simulink model "CarSim_SCANeR_UDP_ACC_THESIS"  (R2019a)
settings: Solver=FixedStepAuto  StartTime=0.0  StopTime=inf  FixedStep=0.001  RelTol=1e-3  EnableMultiTasking=on
undefined symbols (not defined in the file or in its folder): DWORK0, DWORK1
libraries: simulink x14, xpcutilitieslib x2, xpcrtudplib x2, dspnetwork x1
(part 1 of 2)
settings Model: ExtModeTrigDuration=10000  Creator=llacroix  LastModifiedBy=wilkerson.102
settings SolverCC: PositivePriorityOrder=on  InsertRTBMode=Always
settings DataIOCC: ReturnWorkspaceOutputs=off
settings OptimizationCC: UseFloatMulNetSlope=on
settings DebuggingCC: ArithmeticOperatorsInVariantConditions=warning
settings SFSimCC: SimUseLocalCustomCode=off
settings RTWCC: Description=Generic Real-Time Target  RTWUseLocalCustomCode=off  TargetLang=C++
settings CodeAppCC: StateflowObjectComments=on
settings GRTTargetCC: TargetLangStandard=C++03 (ISO)  MatFileLogging=off  MultiInstanceERTCode=on  CodeInterfacePackaging=C++ class

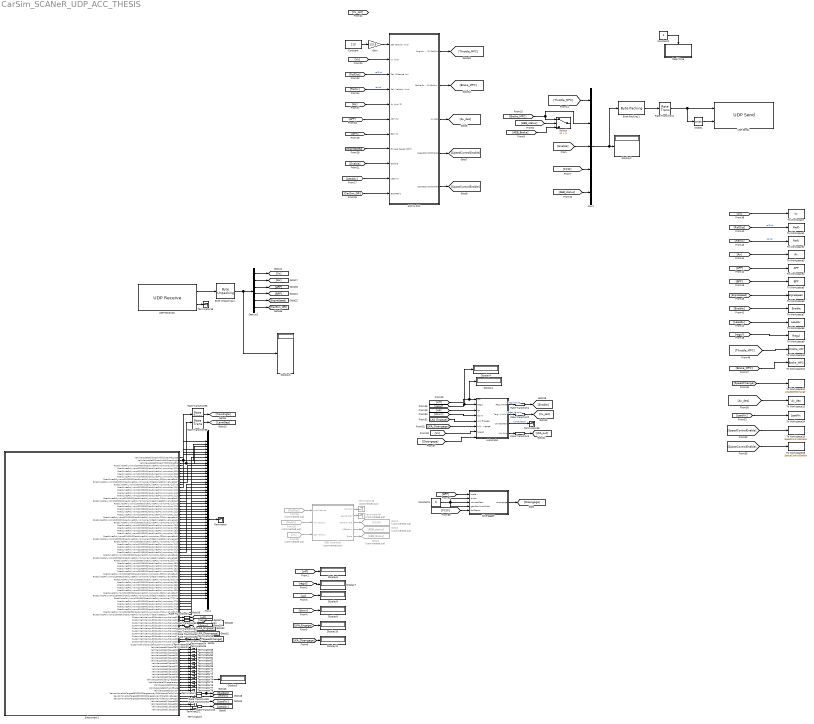
== system CarSim_SCANeR_UDP_ACC_THESIS ==
  ACC & CC1 : Subsystem
  AEB Controller : Subsystem  Commented=on
  Automate : Subsystem
  Byte Packing 1 : xpcutilitieslib/Byte Packing   MaskPackedDataType=uint8  MaskUnpackedDataTypes={'double'}  MaskAlignment=1
  Byte Unpacking 2 : xpcutilitieslib/Byte Unpacking   MaskUnpackedDataTypes={'double'}  MaskUnpackedDataSizes={[6]}  MaskAlignment=1
      settings: SourceProductName=Simulink Real-Time  SourceProductBaseCode=XP
  Constant : Constant  Value=110  VectorParams1D=off
  Constant1 : Constant  Value=0
  Constant2 : Constant
  Demux2 : Demux  Outputs=6
  Disengager : Subsystem
  Display{1..11} (11 alike) : Display
  From16 : From  Commented=on  GotoTag=RelDist
  From35 : From  Commented=on  GotoTag=RelVx
  From36 : From  Commented=on  GotoTag=Vx
  Gain : Gain  Gain=1/3.6
  Goto1 : Goto  Commented=on  GotoTag=FCW
  Goto2 : Goto  Commented=on  GotoTag=AEB_status
  Goto3 : Goto  Commented=on  GotoTag=AEB_Brake
  Mux1 : Mux  Inputs=5
  Mux4 : Mux  Inputs=59
  Rate Transition{1..5,55..64} (15 alike) : RateTransition
  Real-Time : Subsystem
  Subsystem1 : Subsystem
  Switch : Switch  Criteria=u2 > Threshold
  Terminator{,1..3,18,23,53..63,68..78} (28 alike) : Terminator
  Terminator48 : Terminator  Commented=on
  Terminator49 : Terminator  Commented=on
  To Workspace : ToWorkspace  VariableName=Vx  SampleTime=-1
      settings: Save2DSignal=2-D array (concatenate along first dimension)
  To Workspace1 : ToWorkspace  VariableName=RelD  SampleTime=-1
      settings: Save2DSignal=2-D array (concatenate along first dimension)
  To Workspace10 : ToWorkspace  VariableName=Throttle_MPC  SampleTime=-1
      settings: Save2DSignal=2-D array (concatenate along first dimension)
  To Workspace11 : ToWorkspace  VariableName=Brake_MPC  SampleTime=-1
      settings: Save2DSignal=2-D array (concatenate along first dimension)
  To Workspace12 : ToWorkspace  VariableName=LeadSpeedChange  SampleTime=-1
      settings: Save2DSignal=2-D array (concatenate along first dimension)
  To Workspace13 : ToWorkspace  VariableName=Ax_des  SampleTime=-1
      settings: Save2DSignal=2-D array (concatenate along first dimension)
  To Workspace14 : ToWorkspace  VariableName=LeadVx  SampleTime=-1
      settings: Save2DSignal=2-D array (concatenate along first dimension)
  To Workspace15 : ToWorkspace  VariableName=SpeedControlEnable  SampleTime=-1
      settings: Save2DSignal=2-D array (concatenate along first dimension)
  To Workspace16 : ToWorkspace  VariableName=SpaceControlEnable  SampleTime=-1
      settings: Save2DSignal=2-D array (concatenate along first dimension)
  To Workspace2 : ToWorkspace  VariableName=RelV  SampleTime=-1
      settings: Save2DSignal=2-D array (concatenate along first dimension)
  To Workspace3 : ToWorkspace  VariableName=Ax  SampleTime=-1
      settings: Save2DSignal=2-D array (concatenate along first dimension)
  To Workspace4 : ToWorkspace  VariableName=APP  SampleTime=-1
      settings: Save2DSignal=2-D array (concatenate along first dimension)
  To Workspace5 : ToWorkspace  VariableName=BPP  SampleTime=-1
      settings: Save2DSignal=2-D array (concatenate along first dimension)
  To Workspace6 : ToWorkspace  VariableName=EngineSpeed  SampleTime=-1
      settings: Save2DSignal=2-D array (concatenate along first dimension)
  To Workspace7 : ToWorkspace  VariableName=Enable  SampleTime=-1
      settings: Save2DSignal=2-D array (concatenate along first dimension)
  To Workspace8 : ToWorkspace  VariableName=LeadAx  SampleTime=-1
      settings: Save2DSignal=2-D array (concatenate along first dimension)
  To Workspace9 : ToWorkspace  VariableName=Regul  SampleTime=-1
      settings: Save2DSignal=2-D array (concatenate along first dimension)
  UDP Receive2 : xpcrtudplib/UDP Receive  ipAddressVal=Use host-target connection  localPort=25007  rcvWidth=48  rcvFmAny=off  fmAddress=0.0.0.0  rcvMulticast=off  multicastAddress={}  maxUDPQueue=8  sampleTime=0.001
      settings: SourceProductName=Simulink Real-Time
  UDP Send1 : xpcrtudplib/UDP Send  ipAddressVal=Use host-target connection  localPort=-1  toAddress=255.255.255.255  toPort=25004  sampleTime=0.01
      settings: SourceProductName=Simulink Real-Time  SourceProductBaseCode=XP
  Width1 : Width
  wires:
  Automate/2(Target (m/s)) -> Rate Transition2/1  "Target Velocity"
  Automate/1(RegulMode) -> Rate Transition1/1  "RegulMode"
  Automate/3(wantedGear) -> Terminator68/1  "wantedGear"
  Automate/4(LKA Out) -> Rate Transition3/1
  Rate Transition1/1 -> [Enable]
  Rate Transition2/1 -> [Vx_set]
  Rate Transition3/1 -> [LKA_out]
  [off] -> Display1/1, Automate/1(Off)
  [regul] -> Display4/1, Automate/2(Regul)
  [up] -> Automate/3(Up)
  [down] -> Automate/4(Down)
  [LKA_Engage] -> Automate/5(LKA Engage)
  [LKA_Disengage] -> Automate/6(LKA Disengage)
  [Vx] -> Automate/7(Speed)
  [Disengage] -> Automate/8(disengage)
  Rate Transition4/1 -> UDP Send1/1, Width1/1
  Byte Packing 1/1 -> Rate Transition4/1
  Width1/1 -> UDP Send1/2
  [Vx] -> ACC & CC1/2(Vx (m/s))
  [RelDist] -> ACC & CC1/3(Rel. Distance (m))  "relDist"
  [RelVx] -> ACC & CC1/4(Rel. Velocity (m/s))  "relVel"
  [Ax] -> ACC & CC1/5(Ax (m/s^2))
  [APP] -> ACC & CC1/6(APP (%))
  [BPP] -> ACC & CC1/7(BPP (N))
  [EngineSpeed] -> ACC & CC1/8(Eninge Speed (RPM))
  [Enable] -> ACC & CC1/9(Enable)
  [LeadAx] -> ACC & CC1/10(Lead Ax)
  [CarSim_GR] -> ACC & CC1/11(GearRatio)
  ACC & CC1/2(Brake Force (N) CarSim) -> [Brake_MPC]
  ACC & CC1/1(Engine Throttle (%) CarSim) -> [Throttle_MPC]
  Mux1/1 -> Byte Packing 1/1, Display2/1
  [Throttle_MPC] -> Mux1/1
  UDP Receive2/1 -> Byte Unpacking 2/1
  UDP Receive2/2 -> Terminator18/1
  Byte Unpacking 2/1 -> Display3/1, Demux2/1
  Demux2/1 -> [Vx]
  Demux2/2 -> [Ax]
  Demux2/3 -> [APP]
  Demux2/4 -> [BPP]
  Demux2/5 -> [EngineSpeed]
  Demux2/6 -> [CarSim_GR]
  [BPP] -> Disengager/1(brake)
  Constant1/1 -> Disengager/2(clutch), Disengager/4(gearBoxAutoMode), Disengager/3(wantedGear)
  AEB Controller/1(collision) -> Terminator48/1
  From36/1 -> AEB Controller/3(egoVelocity)
  From35/1 -> AEB Controller/2(mioVelocity)
  From16/1 -> AEB Controller/1(mioDistance)
  [FCW] -> Disengager/5(fcwStatus)
  [Enable] -> Mux1/3
  Disengager/1(disengage) -> [Disengage]
  [LKA_Disengage] -> Display11/1
  [LKA_Engage] -> Display10/1
  [down] -> Display9/1
  [up] -> Display8/1
  [regul] -> Display7/1
  [off] -> Display6/1
  Subsystem1/88(SensorMovableTargets[300000]/targetsArray[0]/distanceToCollision) -> Rate Transition63/1
  Subsystem1/89(SensorMovableTargets[300000]/targetsArray[0]/relativeSpeedX) -> Rate Transition64/1
  Subsystem1/1(VehicleUpdate[0]/roadInfo[0]/roadAbscissa) -> Mux4/1
  Subsystem1/2(VehicleUpdate[0]/roadInfo[0]/roadAngle) -> Rate Transition55/1, Mux4/2
  Subsystem1/3(VehicleUpdate[0]/roadInfo[0]/laneGap) -> Rate Transition56/1, Mux4/3
  Subsystem1/4(RoadLinesPolynoms[100000]/roadLinesPolynomsArray[0]/lineId) -> Mux4/4
  Subsystem1/5(RoadLinesPolynoms[100000]/roadLinesPolynomsArray[0]/c0) -> Mux4/5
  Subsystem1/6(RoadLinesPolynoms[100000]/roadLinesPolynomsArray[0]/c1) -> Mux4/6
  Subsystem1/7(RoadLinesPolynoms[100000]/roadLinesPolynomsArray[0]/c2) -> Mux4/7
  Subsystem1/8(RoadLinesPolynoms[100000]/roadLinesPolynomsArray[0]/c3) -> Mux4/8
  Subsystem1/9(RoadLinesPolynoms[100000]/roadLinesPolynomsArray[0]/curvatureRadius) -> Mux4/9
  Subsystem1/10(RoadLinesPolynoms[100000]/roadLinesPolynomsArray[0]/estimatedCurvatureRadius) -> Mux4/10
  Subsystem1/11(RoadLinesPolynoms[100000]/roadLinesPolynomsArray[1]/lineId) -> Mux4/11
  Subsystem1/12(RoadLinesPolynoms[100000]/roadLinesPolynomsArray[1]/c0) -> Mux4/12
  Subsystem1/13(RoadLinesPolynoms[100000]/roadLinesPolynomsArray[1]/c1) -> Mux4/13
  Subsystem1/14(RoadLinesPolynoms[100000]/roadLinesPolynomsArray[1]/c2) -> Mux4/14
  Subsystem1/15(RoadLinesPolynoms[100000]/roadLinesPolynomsArray[1]/c3) -> Mux4/15
  Subsystem1/16(RoadLinesPolynoms[100000]/roadLinesPolynomsArray[1]/curvatureRadius) -> Mux4/16
  Subsystem1/17(RoadLinesPolynoms[100000]/roadLinesPolynomsArray[1]/estimatedCurvatureRadius) -> Mux4/17
  Subsystem1/18(RoadLinesPolynoms[100000]/roadLinesPolynomsArray[2]/lineId) -> Mux4/18
  Subsystem1/19(RoadLinesPolynoms[100000]/roadLinesPolynomsArray[2]/c0) -> Mux4/19
  Subsystem1/20(RoadLinesPolynoms[100000]/roadLinesPolynomsArray[2]/c1) -> Mux4/20
  Subsystem1/21(RoadLinesPolynoms[100000]/roadLinesPolynomsArray[2]/c2) -> Mux4/21
  Subsystem1/22(RoadLinesPolynoms[100000]/roadLinesPolynomsArray[2]/c3) -> Mux4/22
  Subsystem1/23(RoadLinesPolynoms[100000]/roadLinesPolynomsArray[2]/curvatureRadius) -> Mux4/23
  Subsystem1/24(RoadLinesPolynoms[100000]/roadLinesPolynomsArray[2]/estimatedCurvatureRadius) -> Mux4/24
  Subsystem1/25(RoadLinesPolynoms[100000]/roadLinesPolynomsArray[3]/lineId) -> Mux4/25
  Subsystem1/26(RoadLinesPolynoms[100000]/roadLinesPolynomsArray[3]/c0) -> Mux4/26
  Subsystem1/27(RoadLinesPolynoms[100000]/roadLinesPolynomsArray[3]/c1) -> Mux4/27
  Subsystem1/28(RoadLinesPolynoms[100000]/roadLinesPolynomsArray[3]/c2) -> Mux4/28
  Subsystem1/29(RoadLinesPolynoms[100000]/roadLinesPolynomsArray[3]/c3) -> Mux4/29
  Subsystem1/30(RoadLinesPolynoms[100000]/roadLinesPolynomsArray[3]/curvatureRadius) -> Mux4/30
  Subsystem1/31(RoadLinesPolynoms[100000]/roadLinesPolynomsArray[3]/estimatedCurvatureRadius) -> Mux4/31
  Subsystem1/32(RoadLinesPolynoms[100000]/roadLinesPolynomsArray[4]/lineId) -> Mux4/32
  Subsystem1/33(RoadLinesPolynoms[100000]/roadLinesPolynomsArray[4]/c0) -> Mux4/33
  Subsystem1/34(RoadLinesPolynoms[100000]/roadLinesPolynomsArray[4]/c1) -> Mux4/34
  Subsystem1/35(RoadLinesPolynoms[100000]/roadLinesPolynomsArray[4]/c2) -> Mux4/35
  Subsystem1/36(RoadLinesPolynoms[100000]/roadLinesPolynomsArray[4]/c3) -> Mux4/36
  Subsystem1/37(RoadLinesPolynoms[100000]/roadLinesPolynomsArray[4]/curvatureRadius) -> Mux4/37
  Subsystem1/38(RoadLinesPolynoms[100000]/roadLinesPolynomsArray[4]/estimatedCurvatureRadius) -> Mux4/38
  Subsystem1/39(RoadLinesPolynoms[100000]/roadLinesPolynomsArray[5]/lineId) -> Mux4/39
  Subsystem1/40(RoadLinesPolynoms[100000]/roadLinesPolynomsArray[5]/c0) -> Mux4/40
  Subsystem1/41(RoadLinesPolynoms[100000]/roadLinesPolynomsArray[5]/c1) -> Mux4/41
  Subsystem1/42(RoadLinesPolynoms[100000]/roadLinesPolynomsArray[5]/c2) -> Mux4/42
  Subsystem1/43(RoadLinesPolynoms[100000]/roadLinesPolynomsArray[5]/c3) -> Mux4/43
  Subsystem1/44(RoadLinesPolynoms[100000]/roadLinesPolynomsArray[5]/curvatureRadius) -> Mux4/44
  Subsystem1/45(RoadLinesPolynoms[100000]/roadLinesPolynomsArray[5]/estimatedCurvatureRadius) -> Mux4/45
  Subsystem1/46(RoadLinesPolynoms[100000]/roadLinesPolynomsArray[6]/lineId) -> Mux4/46
  Subsystem1/47(RoadLinesPolynoms[100000]/roadLinesPolynomsArray[6]/c0) -> Mux4/47
  Subsystem1/48(RoadLinesPolynoms[100000]/roadLinesPolynomsArray[6]/c1) -> Mux4/48
  Subsystem1/49(RoadLinesPolynoms[100000]/roadLinesPolynomsArray[6]/c2) -> Mux4/49
  Subsystem1/50(RoadLinesPolynoms[100000]/roadLinesPolynomsArray[6]/c3) -> Mux4/50
  Subsystem1/51(RoadLinesPolynoms[100000]/roadLinesPolynomsArray[6]/curvatureRadius) -> Mux4/51
  Subsystem1/52(RoadLinesPolynoms[100000]/roadLinesPolynomsArray[6]/estimatedCurvatureRadius) -> Mux4/52
  Subsystem1/53(RoadLinesPolynoms[100000]/roadLinesPolynomsArray[7]/lineId) -> Mux4/53
  Subsystem1/54(RoadLinesPolynoms[100000]/roadLinesPolynomsArray[7]/c0) -> Mux4/54
  Subsystem1/55(RoadLinesPolynoms[100000]/roadLinesPolynomsArray[7]/c1) -> Mux4/55
  Subsystem1/56(RoadLinesPolynoms[100000]/roadLinesPolynomsArray[7]/c2) -> Mux4/56
  Subsystem1/57(RoadLinesPolynoms[100000]/roadLinesPolynomsArray[7]/c3) -> Mux4/57
  Subsystem1/58(RoadLinesPolynoms[100000]/roadLinesPolynomsArray[7]/curvatureRadius) -> Mux4/58
  Subsystem1/59(RoadLinesPolynoms[100000]/roadLinesPolynomsArray[7]/estimatedCurvatureRadius) -> Mux4/59
  Subsystem1/66(CustomVehicleInput[0]/customInputValues[6]) -> Terminator23/1
  Subsystem1/67(CustomVehicleInput[0]/customInputValues[7]) -> Terminator53/1
  Subsystem1/68(CustomVehicleInput[0]/customInputValues[8]) -> [SpeedChange], Terminator54/1
  Subsystem1/69(CustomVehicleInput[0]/customInputValues[9]) -> Terminator55/1
  Subsystem1/70(CustomVehicleInput[0]/customInputValues[10]) -> Terminator56/1
  Subsystem1/71(VehicleUpdate[0]/speed[0]) -> Terminator57/1
  Subsystem1/72(VehicleUpdate[0]/speed[1]) -> Terminator58/1
  Subsystem1/73(VehicleUpdate[0]/speed[2]) -> Terminator59/1
  Subsystem1/74(VehicleUpdate[0]/speed[3]) -> Terminator60/1
  Subsystem1/75(VehicleUpdate[0]/speed[4]) -> Terminator61/1
  Subsystem1/76(VehicleUpdate[0]/speed[5]) -> Terminator62/1
  Subsystem1/77(VehicleUpdate[0]/accel[0]) -> Terminator63/1
  Subsystem1/78(VehicleUpdate[0]/accel[1]) -> Terminator69/1
  Subsystem1/79(VehicleUpdate[0]/accel[2]) -> Terminator70/1
  Subsystem1/80(VehicleUpdate[0]/accel[3]) -> Terminator71/1
  Subsystem1/81(VehicleUpdate[0]/accel[4]) -> Terminator72/1
  Subsystem1/82(VehicleUpdate[0]/accel[5]) -> Terminator73/1
  Subsystem1/83(VehicleUpdate[0]/engineSpeed) -> Terminator74/1
  Subsystem1/84(VehicleUpdate[0]/accelerator) -> Terminator75/1
  Subsystem1/85(VehicleUpdate[0]/brake) -> Terminator76/1
  Subsystem1/86(VehicleUpdate[0]/handBrake) -> Terminator77/1
  Subsystem1/87(VehicleUpdate[0]/clutch) -> Terminator78/1
  Rate Transition55/1 -> [YawAngle]
  Rate Transition56/1 -> [LaneGap]
  Rate Transition57/1 -> [off]
  Subsystem1/60(CustomVehicleInput[0]/customInputValues[0]) -> Rate Transition57/1
  Subsystem1/61(CustomVehicleInput[0]/customInputValues[1]) -> Rate Transition59/1
  Rate Transition59/1 -> [regul]
  Subsystem1/62(CustomVehicleInput[0]/customInputValues[2]) -> Rate Transition60/1
  Rate Transition60/1 -> [up]
  Subsystem1/63(CustomVehicleInput[0]/customInputValues[3]) -> Rate Transition61/1
  Rate Transition61/1 -> [down]
  Subsystem1/64(CustomVehicleInput[0]/customInputValues[4]) -> Rate Transition62/1
  Rate Transition62/1 -> [LKA_Engage]
  Subsystem1/65(CustomVehicleInput[0]/customInputValues[5]) -> Rate Transition58/1
  Rate Transition58/1 -> [LKA_Disengage]
  Rate Transition63/1 -> [RelDist], Display5/1
  Rate Transition64/1 -> [RelVx]
  Mux4/1 -> Terminator/1
  AEB Controller/2(egoCarStop) -> Terminator49/1
  AEB Controller/3(FCWactivate) -> Goto1/1
  AEB Controller/4(AEBstatus) -> Goto2/1
  AEB Controller/5(Brake) -> Goto3/1
  [Brake_MPC] -> Switch/1, Mux1/2
  [AEB_status] -> Switch/2
  [AEB_Brake] -> Switch/3
  [FCW] -> Mux1/4
  [AEB_status] -> Mux1/5
  Constant/1 -> Gain/1
  Gain/1 -> ACC & CC1/1(Set Velocity (m/s))
  [Vx] -> To Workspace/1
  [RelDist] -> To Workspace1/1  "relDist"
  [RelVx] -> To Workspace2/1  "relVel"
  [Ax] -> To Workspace3/1
  [APP] -> To Workspace4/1
  [BPP] -> To Workspace5/1
  [EngineSpeed] -> To Workspace6/1
  [Enable] -> To Workspace7/1
  [LeadAx] -> To Workspace8/1
  [regul] -> To Workspace9/1
  [Throttle_MPC] -> To Workspace10/1
  [Brake_MPC] -> To Workspace11/1
  Constant2/1 -> Real-Time/Enable
  [SpeedChange] -> To Workspace12/1
  ACC & CC1/3(Ax_des) -> [Ax_des]
  [Ax_des] -> To Workspace13/1
  Subsystem1/93(VehicleUpdate[1]/accel[0]) -> Rate Transition5/1
  Subsystem1/91(VehicleUpdate[1]/speed[0]) -> [LeadVx]
  Subsystem1/90(SensorMovableTargets[300000]/targetsArray[0]/absoluteAccelX) -> Terminator1/1
  Subsystem1/92(VehicleUpdate[1]/speed[1]) -> Terminator2/1
  Subsystem1/94(VehicleUpdate[1]/accel[1]) -> Terminator3/1
  [LeadVx] -> To Workspace14/1
  ACC & CC1/4(SpeedControlEnable) -> [SpeedControlEnable]
  ACC & CC1/5(SpaceControlEnable) -> [SpaceControlEnable]
  [SpeedControlEnable] -> To Workspace15/1
  [SpaceControlEnable] -> To Workspace16/1
  Rate Transition5/1 -> [LeadAx]

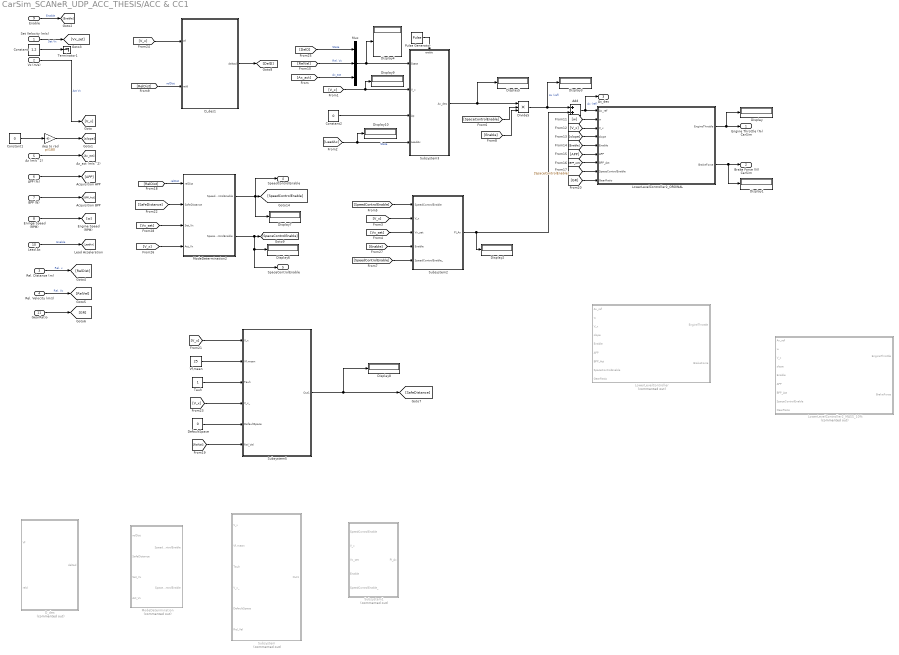
== system CarSim_SCANeR_UDP_ACC_THESIS/ACC & CC1 ==
  Set Velocity (m/s) : Inport
  Vx (m/s) : Inport  Port=2
  Rel. Distance (m) : Inport  Port=3
  Rel. Velocity (m/s) : Inport  Port=4
  Ax (m/s^2) : Inport  Port=5
  APP (%) : Inport  Port=6
  BPP (N) : Inport  Port=7
  Eninge Speed (RPM) : Inport  Port=8
  Enable : Inport  Port=9
  Lead Ax : Inport  Port=10
  GearRatio : Inport  Port=11
  Add : Sum
  Constant : Constant  Value=1.2
  Constant1 : Constant  Value=0
  Constant2 : Constant  Value=0
  D_des : Subsystem  Commented=on  TreatAsAtomicUnit=on
  D_des1 : Subsystem
      mask help: Simulink:masks:GenSFuncDesc_MD
      mask Help: eval('feval(''rtwprivate'',''rtwhelpview'',''rtw_sfcn_block'')');
  DefaultSpace : Constant  Value=0
  Display{,1..10} (11 alike) : Display
  Divide5 : Product  Inputs=***
  LowerLevelController : Subsystem  Commented=on  TreatAsAtomicUnit=on
  LowerLevelController2_MASS_10% : Subsystem  Commented=on
      mask help: Simulink:masks:GenSFuncDesc_MD
      mask Help: eval('feval(''rtwprivate'',''rtwhelpview'',''rtw_sfcn_block'')');
  LowerLevelController2_ORGINAL : Subsystem
      mask help: Simulink:masks:GenSFuncDesc_MD
      mask Help: eval('feval(''rtwprivate'',''rtwhelpview'',''rtw_sfcn_block'')');
  ModeDetermination : Subsystem  Commented=on  TreatAsAtomicUnit=on
  ModeDetermination2 : Subsystem
      mask help: Simulink:masks:GenSFuncDesc_MD
      mask Help: eval('feval(''rtwprivate'',''rtwhelpview'',''rtw_sfcn_block'')');
  Mux : Mux  Inputs=3
  Pulse Generator : DiscretePulseGenerator  PulseType=Time based  Period=0.05  PulseWidth=10
  Subsystem : Subsystem  Commented=on  TreatAsAtomicUnit=on
  Subsystem1 : Subsystem  Commented=on  TreatAsAtomicUnit=on
  Subsystem2 : Subsystem
      mask help: Simulink:masks:GenSFuncDesc_MD
      mask Help: eval('feval(''rtwprivate'',''rtwhelpview'',''rtw_sfcn_block'')');
  Subsystem3 : Subsystem
  Subsystem5 : Subsystem
      mask help: Simulink:masks:GenSFuncDesc_MD
      mask Help: eval('feval(''rtwprivate'',''rtwhelpview'',''rtw_sfcn_block'')');
  Tauh : Constant
  Terminator1 : Terminator
  Vf,mean : Constant  Value=25
  deg to rad : Gain  Gain=pi/180
  Engine Throttle (%) CarSim : Outport  VectorParamsAs1DForOutWhenUnconnected=on
  Brake Force (N) CarSim : Outport  Port=2  VectorParamsAs1DForOutWhenUnconnected=on
  Ax_des : Outport  Port=3  VectorParamsAs1DForOutWhenUnconnected=on
  SpeedControlEnable : Outport  Port=4  VectorParamsAs1DForOutWhenUnconnected=on
  SpaceControlEnable : Outport  Port=5  VectorParamsAs1DForOutWhenUnconnected=on
  wires:
  [Ax_act] -> Mux/3  "Ax_act"
  [DelD] -> Mux/1  "State"
  GearRatio/1 -> [GR]
  Rel. Velocity (m/s)/1 -> [RelVel]  "Rel. Vx"
  Rel. Distance (m)/1 -> [RelDist]  "Rel. x"
  [Enable] -> Divide5/3
  [SpaceControlEnable] -> Divide5/2
  Divide5/1 -> Add/1, Display3/1  "Ax (ref)"
  Enable/1 -> [Enable]  "Enable"
  APP (%)/1 -> [APP]
  Ax (m/s^2)/1 -> [Ax_act]
  Vx (m/s)/1 -> [V_x]  "Act Vx"
  [RelVel] -> Mux/2  "Rel. Vx"
  Eninge Speed (RPM)/1 -> [w]
  BPP (N)/1 -> [BPP_Act]
  Constant1/1 -> deg to rad/1
  Lead Ax/1 -> [LeadAx]  "Enable"
  Set Velocity (m/s)/1 -> [Vx_set]  "Set Vx"
  Constant/1 -> Terminator1/1
  ModeDetermination2/1(SpeedControlEnable) -> SpeedControlEnable/1, Display7/1, [SpeedControlEnable]
  Subsystem2/1(PI_Ax) -> Display2/1, Add/2
  ModeDetermination2/2(SpaceControlEnable) -> SpaceControlEnable/1, Display6/1, [SpaceControlEnable]
  Subsystem3/1(Ax_des) -> Display5/1, Divide5/1
  Mux/1 -> Display4/1, Subsystem3/1(State)
  [V_x] -> Display9/1, Subsystem3/2(V_x)
  Constant2/1 -> Subsystem3/3(Ap)
  [LeadAx] -> Display10/1, Subsystem3/4(LeadAx)  "State"
  Pulse Generator/1 -> Subsystem3/Enable
  [SpeedControlEnable] -> Subsystem2/1(SpeedControlEnable)
  [V_x] -> Subsystem2/2(V_x)
  [Vx_set] -> Subsystem2/3(Vx_set)
  [Enable] -> Subsystem2/4(Enable)
  [SpeedControlEnable] -> Subsystem2/5(SpeedControlEnable_)
  [RelDist] -> ModeDetermination2/1(relDist)  "relDist"
  D_des1/1(deltad) -> [DelD]
  [RelDist] -> D_des1/2(reld)  "relDist"
  [V_x] -> D_des1/1("Vf ")
  [SafeDistance] -> ModeDetermination2/2(SafeDistance)
  [V_x] -> ModeDetermination2/4(Act_Vx)
  [Vx_set] -> ModeDetermination2/3(Set_Vx)
  [RelVel] -> Subsystem5/6(Rel_Vel)
  [V_x] -> Subsystem5/4(V_x_)
  DefaultSpace/1 -> Subsystem5/5(DefaultSpace)
  Tauh/1 -> Subsystem5/3(Tauh)
  Vf,mean/1 -> Subsystem5/2(Vf,mean)
  [V_x] -> Subsystem5/1(V_x)
  Subsystem5/1(Out1) -> Display8/1, [SafeDistance]
  Add/1 -> LowerLevelController2_ORGINAL/1(Ax_ref), Ax_des/1  "Ax (ref)"
  [GR] -> LowerLevelController2_ORGINAL/9(GearRatio)
  [SpaceControlEnable] -> LowerLevelController2_ORGINAL/8(SpaceControlEnable)
  [BPP_Act] -> LowerLevelController2_ORGINAL/7(BPP_Act)
  [APP] -> LowerLevelController2_ORGINAL/6(APP)
  [Enable] -> LowerLevelController2_ORGINAL/5(Enable)
  [slope] -> LowerLevelController2_ORGINAL/4(slope)
  [V_x] -> LowerLevelController2_ORGINAL/3(V_x)
  [w] -> LowerLevelController2_ORGINAL/2(w)
  LowerLevelController2_ORGINAL/1(EngineThrottle) -> Display/1, Engine Throttle (%) CarSim/1
  LowerLevelController2_ORGINAL/2(BrakeForce) -> Display1/1, Brake Force (N) CarSim/1
  deg to rad/1 -> [slope]

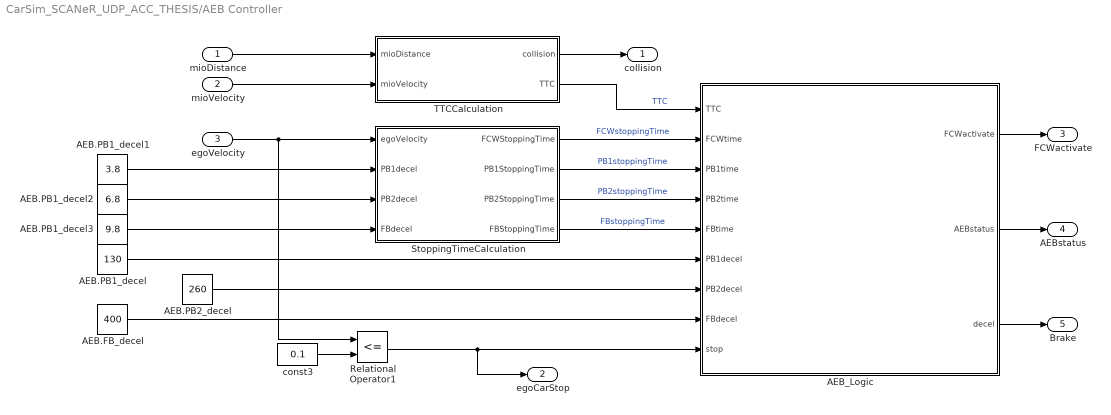
== system CarSim_SCANeR_UDP_ACC_THESIS/AEB Controller ==
  mioDistance : Inport
  mioVelocity : Inport  Port=2
  egoVelocity : Inport  Port=3
  AEB.FB_decel : Constant  Value=400
  AEB.PB1_decel : Constant  Value=130
  AEB.PB1_decel1 : Constant  Value=3.8
  AEB.PB1_decel2 : Constant  Value=6.8
  AEB.PB1_decel3 : Constant  Value=9.8
  AEB.PB2_decel : Constant  Value=260
  AEB_Logic : Stateflow chart  TreatAsAtomicUnit=on
  Relational Operator1 : RelationalOperator  Operator=<=  OutDataTypeStr=boolean  RndMeth=Simplest
  StoppingTimeCalculation : Subsystem
  TTCCalculation : Subsystem
  const3 : Constant  Value=0.1  SampleTime=-1
  collision : Outport
  egoCarStop : Outport  Port=2
  FCWactivate : Outport  Port=3
  AEBstatus : Outport  Port=4
  Brake : Outport  Port=5
  wires:
  TTCCalculation/2(TTC) -> AEB_Logic/1(TTC)  "TTC"
  TTCCalculation/1(collision) -> collision/1
  mioVelocity/1 -> TTCCalculation/2(mioVelocity)
  mioDistance/1 -> TTCCalculation/1(mioDistance)
  AEB_Logic/1(FCWactivate) -> FCWactivate/1
  StoppingTimeCalculation/1(FCWStoppingTime) -> AEB_Logic/2(FCWtime)  "FCWstoppingTime"
  StoppingTimeCalculation/4(FBStoppingTime) -> AEB_Logic/5(FBtime)  "FBstoppingTime"
  StoppingTimeCalculation/2(PB1StoppingTime) -> AEB_Logic/3(PB1time)  "PB1stoppingTime"
  StoppingTimeCalculation/3(PB2StoppingTime) -> AEB_Logic/4(PB2time)  "PB2stoppingTime"
  AEB.PB1_decel/1 -> AEB_Logic/6(PB1decel)
  Relational Operator1/1 -> AEB_Logic/9(stop), egoCarStop/1
  const3/1 -> Relational Operator1/2
  AEB.FB_decel/1 -> AEB_Logic/8(FBdecel)
  AEB.PB2_decel/1 -> AEB_Logic/7(PB2decel)
  egoVelocity/1 -> Relational Operator1/1, StoppingTimeCalculation/1(egoVelocity)
  AEB_Logic/2(AEBstatus) -> AEBstatus/1
  AEB_Logic/3(decel) -> Brake/1
  AEB.PB1_decel1/1 -> StoppingTimeCalculation/2(PB1decel)
  AEB.PB1_decel2/1 -> StoppingTimeCalculation/3(PB2decel)
  AEB.PB1_decel3/1 -> StoppingTimeCalculation/4(FBdecel)

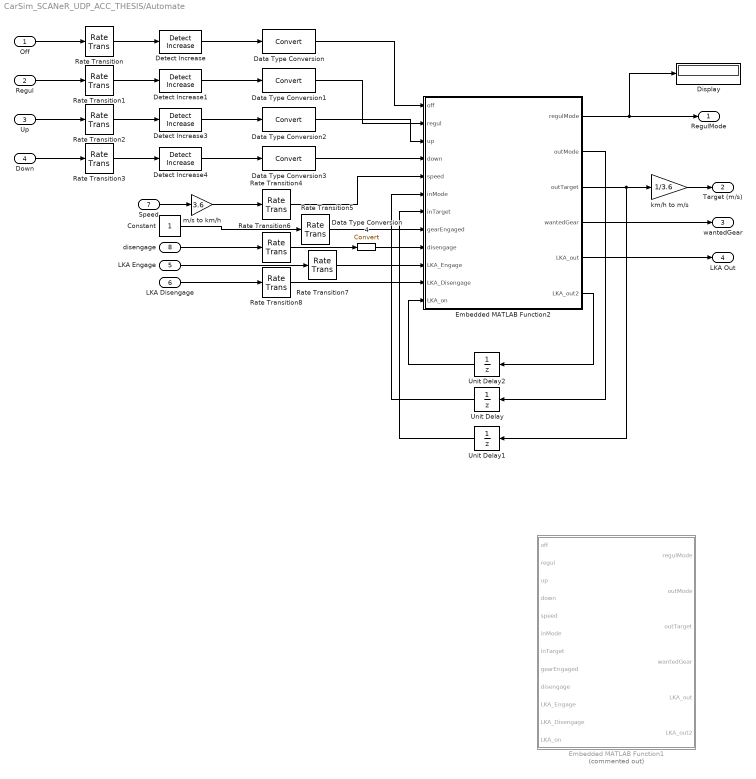
== system CarSim_SCANeR_UDP_ACC_THESIS/Automate ==
  Off : Inport  PortDimensions=1
  Regul : Inport  Port=2  PortDimensions=1
  Up : Inport  Port=3  PortDimensions=1
  Down : Inport  Port=4  PortDimensions=1
  LKA Engage : Inport  Port=5  PortDimensions=1
  LKA Disengage : Inport  Port=6  PortDimensions=1
  Speed : Inport  Port=7  PortDimensions=1
  disengage : Inport  Port=8  PortDimensions=1
  Constant : Constant
  Data Type Conversion{,1..4} (5 alike) : DataTypeConversion
  Detect Increase{,1,3..4} (4 alike) : simulink/Logic and Bit Operations/Detect Increase  vinit=0.0  OutDataTypeStr=uint8
  Display : Display
  Embedded MATLAB Function1 : MATLAB Function  Commented=on  TreatAsAtomicUnit=on
  Embedded MATLAB Function2 : Subsystem
      mask help: Simulink:masks:GenSFuncDesc_MD
      mask Help: eval('feval(''rtwprivate'',''rtwhelpview'',''rtw_sfcn_block'')');
  Rate Transition{,1..8} (9 alike) : RateTransition
  Unit Delay : UnitDelay  SampleTime=-1
  Unit Delay1 : UnitDelay  SampleTime=-1
  Unit Delay2 : UnitDelay  SampleTime=-1
  km/h to m/s : Gain  Gain=1/3.6
  m/s to km/h : Gain  Gain=3.6
  RegulMode : Outport
  Target (m/s) : Outport  Port=2
  wantedGear : Outport  Port=3
  LKA Out : Outport  Port=4
  wires:
  Rate Transition8/1 -> Embedded MATLAB Function2/11(LKA_Disengage)
  Rate Transition7/1 -> Embedded MATLAB Function2/10(LKA_Engage)
  Rate Transition6/1 -> Data Type Conversion4/1
  Rate Transition5/1 -> Embedded MATLAB Function2/8(gearEngaged)
  Rate Transition4/1 -> Embedded MATLAB Function2/5(speed)
  Rate Transition3/1 -> Detect Increase4/1
  Rate Transition2/1 -> Detect Increase3/1
  Rate Transition1/1 -> Detect Increase1/1
  Rate Transition/1 -> Detect Increase/1
  Data Type Conversion3/1 -> Embedded MATLAB Function2/4(down)
  Data Type Conversion2/1 -> Embedded MATLAB Function2/3(up)
  Data Type Conversion1/1 -> Embedded MATLAB Function2/2(regul)
  Data Type Conversion/1 -> Embedded MATLAB Function2/1(off)
  Unit Delay2/1 -> Embedded MATLAB Function2/12(LKA_on)
  Embedded MATLAB Function2/6(LKA_out2) -> Unit Delay2/1
  disengage/1 -> Rate Transition6/1
  Constant/1 -> Rate Transition5/1
  Speed/1 -> m/s to km/h/1
  LKA Disengage/1 -> Rate Transition8/1
  LKA Engage/1 -> Rate Transition7/1
  Embedded MATLAB Function2/5(LKA_out) -> LKA Out/1
  Off/1 -> Rate Transition/1
  Down/1 -> Rate Transition3/1
  Up/1 -> Rate Transition2/1
  Regul/1 -> Rate Transition1/1
  km/h to m/s/1 -> Target (m/s)/1
  Detect Increase/1 -> Data Type Conversion/1
  Detect Increase1/1 -> Data Type Conversion1/1
  Detect Increase3/1 -> Data Type Conversion2/1
  Detect Increase4/1 -> Data Type Conversion3/1
  m/s to km/h/1 -> Rate Transition4/1
  Embedded MATLAB Function2/4(wantedGear) -> wantedGear/1
  Embedded MATLAB Function2/3(outTarget) -> km/h to m/s/1, Unit Delay1/1
  Unit Delay/1 -> Embedded MATLAB Function2/6(inMode)
  Embedded MATLAB Function2/2(outMode) -> Unit Delay/1
  Unit Delay1/1 -> Embedded MATLAB Function2/7(inTarget)
  Embedded MATLAB Function2/1(regulMode) -> Display/1, RegulMode/1
  Data Type Conversion4/1 -> Embedded MATLAB Function2/9(disengage)

== system CarSim_SCANeR_UDP_ACC_THESIS/Disengager ==
  brake : Inport
  clutch : Inport  Port=2
  wantedGear : Inport  Port=3
  gearBoxAutoMode : Inport  Port=4
  fcwStatus : Inport  Port=5
  Compare To Constant1 : simulink/Logic and Bit Operations/Compare To Constant  relop=>=  const=.1  OutDataTypeStr=uint8  ZeroCross=off
  Compare To Constant2 : simulink/Logic and Bit Operations/Compare To Constant  relop=>=  const=.1  OutDataTypeStr=uint8  ZeroCross=off
  Compare To Constant3 : simulink/Logic and Bit Operations/Compare To Constant  relop=>=  const=.1  OutDataTypeStr=uint8  ZeroCross=off
  Detect Change : simulink/Logic and Bit Operations/Detect Change  vinit=0  OutDataTypeStr=uint8
  Detect Change1 : simulink/Logic and Bit Operations/Detect Change  vinit=0  OutDataTypeStr=uint8
  Logical Operator : Logic  Operator=OR  Inputs=5  AllPortsSameDT=off  OutDataTypeStr=boolean
  disengage : Outport
  wires:
  Compare To Constant3/1 -> Logical Operator/5
  fcwStatus/1 -> Compare To Constant3/1
  Detect Change1/1 -> Logical Operator/4
  gearBoxAutoMode/1 -> Detect Change1/1
  Logical Operator/1 -> disengage/1
  Detect Change/1 -> Logical Operator/3
  Compare To Constant2/1 -> Logical Operator/2
  Compare To Constant1/1 -> Logical Operator/1
  wantedGear/1 -> Detect Change/1
  clutch/1 -> Compare To Constant2/1
  brake/1 -> Compare To Constant1/1

== system CarSim_SCANeR_UDP_ACC_THESIS/Real-Time ==
  Enable : EnablePort
  Terminator1 : Terminator
  Timer for Real-Time : S-Function  FunctionName=sfun_rttime  Parameters=1  SFunctionDeploymentMode=off  EnableBusSupport=off
  wires:
  Timer for Real-Time/1 -> Terminator1/1

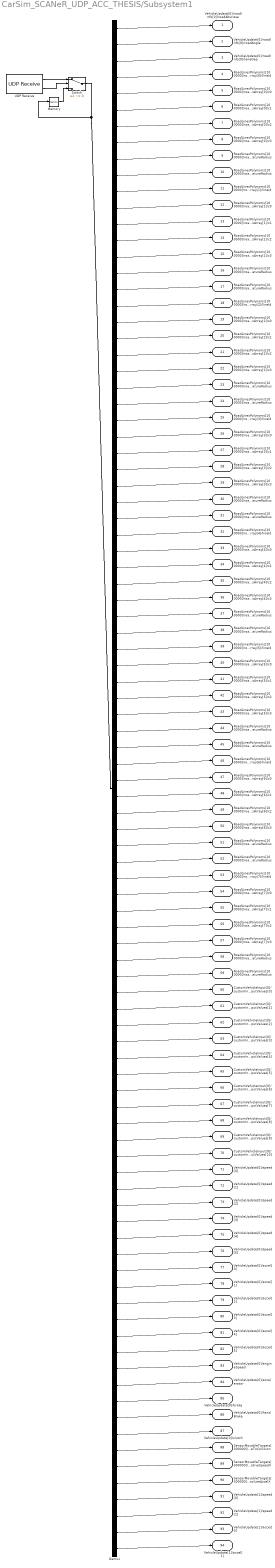
== system CarSim_SCANeR_UDP_ACC_THESIS/Subsystem1 ==
  Demux : Demux  Outputs=94
  Memory : Memory  InheritSampleTime=on
  Switch : Switch  Criteria=u2 ~= 0
  UDP Receive : dspnetwork/UDP Receive  localURL='0.0.0.0'  localPort=8194  remoteURL='0.0.0.0'  remotePort=-1  recvBufferSize=752  dims=94  signalDatatype=double  isComplex=off  isVarSize=off  showBlockingTime=on  blockingTime=0  sampletime=0.01  blockPlatform=HOST
      settings: SourceProductName=Simulink
  VehicleUpdate[0]/roadInfo[0]/roadAbscissa : Outport
  VehicleUpdate[0]/roadInfo[0]/roadAngle : Outport  Port=2
  VehicleUpdate[0]/roadInfo[0]/laneGap : Outport  Port=3
  RoadLinesPolynoms[100000]/roadLinesPolynomsArray[0]/lineId : Outport  Port=4
  RoadLinesPolynoms[100000]/roadLinesPolynomsArray[0]/c0 : Outport  Port=5
  RoadLinesPolynoms[100000]/roadLinesPolynomsArray[0]/c1 : Outport  Port=6
  RoadLinesPolynoms[100000]/roadLinesPolynomsArray[0]/c2 : Outport  Port=7
  RoadLinesPolynoms[100000]/roadLinesPolynomsArray[0]/c3 : Outport  Port=8
  RoadLinesPolynoms[100000]/roadLinesPolynomsArray[0]/curvatureRadius : Outport  Port=9
  RoadLinesPolynoms[100000]/roadLinesPolynomsArray[0]/estimatedCurvatureRadius : Outport  Port=10
  RoadLinesPolynoms[100000]/roadLinesPolynomsArray[1]/lineId : Outport  Port=11
  RoadLinesPolynoms[100000]/roadLinesPolynomsArray[1]/c0 : Outport  Port=12
  RoadLinesPolynoms[100000]/roadLinesPolynomsArray[1]/c1 : Outport  Port=13
  RoadLinesPolynoms[100000]/roadLinesPolynomsArray[1]/c2 : Outport  Port=14
  RoadLinesPolynoms[100000]/roadLinesPolynomsArray[1]/c3 : Outport  Port=15
  RoadLinesPolynoms[100000]/roadLinesPolynomsArray[1]/curvatureRadius : Outport  Port=16
  RoadLinesPolynoms[100000]/roadLinesPolynomsArray[1]/estimatedCurvatureRadius : Outport  Port=17
  RoadLinesPolynoms[100000]/roadLinesPolynomsArray[2]/lineId : Outport  Port=18
  RoadLinesPolynoms[100000]/roadLinesPolynomsArray[2]/c0 : Outport  Port=19
  RoadLinesPolynoms[100000]/roadLinesPolynomsArray[2]/c1 : Outport  Port=20
  RoadLinesPolynoms[100000]/roadLinesPolynomsArray[2]/c2 : Outport  Port=21
  RoadLinesPolynoms[100000]/roadLinesPolynomsArray[2]/c3 : Outport  Port=22
  RoadLinesPolynoms[100000]/roadLinesPolynomsArray[2]/curvatureRadius : Outport  Port=23
  RoadLinesPolynoms[100000]/roadLinesPolynomsArray[2]/estimatedCurvatureRadius : Outport  Port=24
  RoadLinesPolynoms[100000]/roadLinesPolynomsArray[3]/lineId : Outport  Port=25
  RoadLinesPolynoms[100000]/roadLinesPolynomsArray[3]/c0 : Outport  Port=26
  RoadLinesPolynoms[100000]/roadLinesPolynomsArray[3]/c1 : Outport  Port=27
  RoadLinesPolynoms[100000]/roadLinesPolynomsArray[3]/c2 : Outport  Port=28
  RoadLinesPolynoms[100000]/roadLinesPolynomsArray[3]/c3 : Outport  Port=29
  RoadLinesPolynoms[100000]/roadLinesPolynomsArray[3]/curvatureRadius : Outport  Port=30
  RoadLinesPolynoms[100000]/roadLinesPolynomsArray[3]/estimatedCurvatureRadius : Outport  Port=31
  RoadLinesPolynoms[100000]/roadLinesPolynomsArray[4]/lineId : Outport  Port=32
  RoadLinesPolynoms[100000]/roadLinesPolynomsArray[4]/c0 : Outport  Port=33
  RoadLinesPolynoms[100000]/roadLinesPolynomsArray[4]/c1 : Outport  Port=34
  RoadLinesPolynoms[100000]/roadLinesPolynomsArray[4]/c2 : Outport  Port=35
  RoadLinesPolynoms[100000]/roadLinesPolynomsArray[4]/c3 : Outport  Port=36
  RoadLinesPolynoms[100000]/roadLinesPolynomsArray[4]/curvatureRadius : Outport  Port=37
  RoadLinesPolynoms[100000]/roadLinesPolynomsArray[4]/estimatedCurvatureRadius : Outport  Port=38
  RoadLinesPolynoms[100000]/roadLinesPolynomsArray[5]/lineId : Outport  Port=39
  RoadLinesPolynoms[100000]/roadLinesPolynomsArray[5]/c0 : Outport  Port=40
  RoadLinesPolynoms[100000]/roadLinesPolynomsArray[5]/c1 : Outport  Port=41
  RoadLinesPolynoms[100000]/roadLinesPolynomsArray[5]/c2 : Outport  Port=42
  RoadLinesPolynoms[100000]/roadLinesPolynomsArray[5]/c3 : Outport  Port=43
  RoadLinesPolynoms[100000]/roadLinesPolynomsArray[5]/curvatureRadius : Outport  Port=44
  RoadLinesPolynoms[100000]/roadLinesPolynomsArray[5]/estimatedCurvatureRadius : Outport  Port=45
  RoadLinesPolynoms[100000]/roadLinesPolynomsArray[6]/lineId : Outport  Port=46
  RoadLinesPolynoms[100000]/roadLinesPolynomsArray[6]/c0 : Outport  Port=47
  RoadLinesPolynoms[100000]/roadLinesPolynomsArray[6]/c1 : Outport  Port=48
  RoadLinesPolynoms[100000]/roadLinesPolynomsArray[6]/c2 : Outport  Port=49
  RoadLinesPolynoms[100000]/roadLinesPolynomsArray[6]/c3 : Outport  Port=50
  RoadLinesPolynoms[100000]/roadLinesPolynomsArray[6]/curvatureRadius : Outport  Port=51
  RoadLinesPolynoms[100000]/roadLinesPolynomsArray[6]/estimatedCurvatureRadius : Outport  Port=52
  RoadLinesPolynoms[100000]/roadLinesPolynomsArray[7]/lineId : Outport  Port=53
  RoadLinesPolynoms[100000]/roadLinesPolynomsArray[7]/c0 : Outport  Port=54
  RoadLinesPolynoms[100000]/roadLinesPolynomsArray[7]/c1 : Outport  Port=55
  RoadLinesPolynoms[100000]/roadLinesPolynomsArray[7]/c2 : Outport  Port=56
  RoadLinesPolynoms[100000]/roadLinesPolynomsArray[7]/c3 : Outport  Port=57
  RoadLinesPolynoms[100000]/roadLinesPolynomsArray[7]/curvatureRadius : Outport  Port=58
  RoadLinesPolynoms[100000]/roadLinesPolynomsArray[7]/estimatedCurvatureRadius : Outport  Port=59
  CustomVehicleInput[0]/customInputValues[0] : Outport  Port=60
  CustomVehicleInput[0]/customInputValues[1] : Outport  Port=61
  CustomVehicleInput[0]/customInputValues[2] : Outport  Port=62
  CustomVehicleInput[0]/customInputValues[3] : Outport  Port=63
  CustomVehicleInput[0]/customInputValues[4] : Outport  Port=64
  CustomVehicleInput[0]/customInputValues[5] : Outport  Port=65
  CustomVehicleInput[0]/customInputValues[6] : Outport  Port=66
  CustomVehicleInput[0]/customInputValues[7] : Outport  Port=67
  CustomVehicleInput[0]/customInputValues[8] : Outport  Port=68
  CustomVehicleInput[0]/customInputValues[9] : Outport  Port=69
  CustomVehicleInput[0]/customInputValues[10] : Outport  Port=70
  VehicleUpdate[0]/speed[0] : Outport  Port=71
  VehicleUpdate[0]/speed[1] : Outport  Port=72
  VehicleUpdate[0]/speed[2] : Outport  Port=73
  VehicleUpdate[0]/speed[3] : Outport  Port=74
  VehicleUpdate[0]/speed[4] : Outport  Port=75
  VehicleUpdate[0]/speed[5] : Outport  Port=76
  VehicleUpdate[0]/accel[0] : Outport  Port=77
  VehicleUpdate[0]/accel[1] : Outport  Port=78
  VehicleUpdate[0]/accel[2] : Outport  Port=79
  VehicleUpdate[0]/accel[3] : Outport  Port=80
  VehicleUpdate[0]/accel[4] : Outport  Port=81
  VehicleUpdate[0]/accel[5] : Outport  Port=82
  VehicleUpdate[0]/engineSpeed : Outport  Port=83
  VehicleUpdate[0]/accelerator : Outport  Port=84
  VehicleUpdate[0]/brake : Outport  Port=85
  VehicleUpdate[0]/handBrake : Outport  Port=86
  VehicleUpdate[0]/clutch : Outport  Port=87
  SensorMovableTargets[300000]/targetsArray[0]/distanceToCollision : Outport  Port=88
  SensorMovableTargets[300000]/targetsArray[0]/relativeSpeedX : Outport  Port=89
  SensorMovableTargets[300000]/targetsArray[0]/absoluteAccelX : Outport  Port=90
  VehicleUpdate[1]/speed[0] : Outport  Port=91
  VehicleUpdate[1]/speed[1] : Outport  Port=92
  VehicleUpdate[1]/accel[0] : Outport  Port=93
  VehicleUpdate[1]/accel[1] : Outport  Port=94
  wires:
  Memory/1 -> Switch/3
  Switch/1 -> Demux/1, Memory/1
  UDP Receive/2 -> Switch/2
  Demux/94 -> VehicleUpdate[1]/accel[1]/1
  Demux/93 -> VehicleUpdate[1]/accel[0]/1
  Demux/92 -> VehicleUpdate[1]/speed[1]/1
  Demux/91 -> VehicleUpdate[1]/speed[0]/1
  Demux/90 -> SensorMovableTargets[300000]/targetsArray[0]/absoluteAccelX/1
  Demux/89 -> SensorMovableTargets[300000]/targetsArray[0]/relativeSpeedX/1
  Demux/88 -> SensorMovableTargets[300000]/targetsArray[0]/distanceToCollision/1
  Demux/87 -> VehicleUpdate[0]/clutch/1
  Demux/86 -> VehicleUpdate[0]/handBrake/1
  Demux/85 -> VehicleUpdate[0]/brake/1
  Demux/84 -> VehicleUpdate[0]/accelerator/1
  Demux/83 -> VehicleUpdate[0]/engineSpeed/1
  Demux/82 -> VehicleUpdate[0]/accel[5]/1
  Demux/81 -> VehicleUpdate[0]/accel[4]/1
  Demux/80 -> VehicleUpdate[0]/accel[3]/1
  Demux/79 -> VehicleUpdate[0]/accel[2]/1
  Demux/78 -> VehicleUpdate[0]/accel[1]/1
  Demux/77 -> VehicleUpdate[0]/accel[0]/1
  Demux/76 -> VehicleUpdate[0]/speed[5]/1
  Demux/75 -> VehicleUpdate[0]/speed[4]/1
  Demux/74 -> VehicleUpdate[0]/speed[3]/1
  Demux/73 -> VehicleUpdate[0]/speed[2]/1
  Demux/72 -> VehicleUpdate[0]/speed[1]/1
  Demux/71 -> VehicleUpdate[0]/speed[0]/1
  Demux/70 -> CustomVehicleInput[0]/customInputValues[10]/1
  Demux/69 -> CustomVehicleInput[0]/customInputValues[9]/1
  Demux/68 -> CustomVehicleInput[0]/customInputValues[8]/1
  Demux/67 -> CustomVehicleInput[0]/customInputValues[7]/1
  Demux/66 -> CustomVehicleInput[0]/customInputValues[6]/1
  Demux/65 -> CustomVehicleInput[0]/customInputValues[5]/1
  Demux/64 -> CustomVehicleInput[0]/customInputValues[4]/1
  Demux/63 -> CustomVehicleInput[0]/customInputValues[3]/1
  Demux/62 -> CustomVehicleInput[0]/customInputValues[2]/1
  Demux/61 -> CustomVehicleInput[0]/customInputValues[1]/1
  Demux/60 -> CustomVehicleInput[0]/customInputValues[0]/1
  Demux/59 -> RoadLinesPolynoms[100000]/roadLinesPolynomsArray[7]/estimatedCurvatureRadius/1
  Demux/58 -> RoadLinesPolynoms[100000]/roadLinesPolynomsArray[7]/curvatureRadius/1
  Demux/57 -> RoadLinesPolynoms[100000]/roadLinesPolynomsArray[7]/c3/1
  Demux/56 -> RoadLinesPolynoms[100000]/roadLinesPolynomsArray[7]/c2/1
  Demux/55 -> RoadLinesPolynoms[100000]/roadLinesPolynomsArray[7]/c1/1
  Demux/54 -> RoadLinesPolynoms[100000]/roadLinesPolynomsArray[7]/c0/1
  Demux/53 -> RoadLinesPolynoms[100000]/roadLinesPolynomsArray[7]/lineId/1
  Demux/52 -> RoadLinesPolynoms[100000]/roadLinesPolynomsArray[6]/estimatedCurvatureRadius/1
  Demux/51 -> RoadLinesPolynoms[100000]/roadLinesPolynomsArray[6]/curvatureRadius/1
  Demux/50 -> RoadLinesPolynoms[100000]/roadLinesPolynomsArray[6]/c3/1
  Demux/49 -> RoadLinesPolynoms[100000]/roadLinesPolynomsArray[6]/c2/1
  Demux/48 -> RoadLinesPolynoms[100000]/roadLinesPolynomsArray[6]/c1/1
  Demux/47 -> RoadLinesPolynoms[100000]/roadLinesPolynomsArray[6]/c0/1
  Demux/46 -> RoadLinesPolynoms[100000]/roadLinesPolynomsArray[6]/lineId/1
  Demux/45 -> RoadLinesPolynoms[100000]/roadLinesPolynomsArray[5]/estimatedCurvatureRadius/1
  Demux/44 -> RoadLinesPolynoms[100000]/roadLinesPolynomsArray[5]/curvatureRadius/1
  Demux/43 -> RoadLinesPolynoms[100000]/roadLinesPolynomsArray[5]/c3/1
  Demux/42 -> RoadLinesPolynoms[100000]/roadLinesPolynomsArray[5]/c2/1
  Demux/41 -> RoadLinesPolynoms[100000]/roadLinesPolynomsArray[5]/c1/1
  Demux/40 -> RoadLinesPolynoms[100000]/roadLinesPolynomsArray[5]/c0/1
  Demux/39 -> RoadLinesPolynoms[100000]/roadLinesPolynomsArray[5]/lineId/1
  Demux/38 -> RoadLinesPolynoms[100000]/roadLinesPolynomsArray[4]/estimatedCurvatureRadius/1
  Demux/37 -> RoadLinesPolynoms[100000]/roadLinesPolynomsArray[4]/curvatureRadius/1
  Demux/36 -> RoadLinesPolynoms[100000]/roadLinesPolynomsArray[4]/c3/1
  Demux/35 -> RoadLinesPolynoms[100000]/roadLinesPolynomsArray[4]/c2/1
  Demux/34 -> RoadLinesPolynoms[100000]/roadLinesPolynomsArray[4]/c1/1
  Demux/33 -> RoadLinesPolynoms[100000]/roadLinesPolynomsArray[4]/c0/1
  Demux/32 -> RoadLinesPolynoms[100000]/roadLinesPolynomsArray[4]/lineId/1
  Demux/31 -> RoadLinesPolynoms[100000]/roadLinesPolynomsArray[3]/estimatedCurvatureRadius/1
  Demux/30 -> RoadLinesPolynoms[100000]/roadLinesPolynomsArray[3]/curvatureRadius/1
  Demux/29 -> RoadLinesPolynoms[100000]/roadLinesPolynomsArray[3]/c3/1
  Demux/28 -> RoadLinesPolynoms[100000]/roadLinesPolynomsArray[3]/c2/1
  Demux/27 -> RoadLinesPolynoms[100000]/roadLinesPolynomsArray[3]/c1/1
  Demux/26 -> RoadLinesPolynoms[100000]/roadLinesPolynomsArray[3]/c0/1
  Demux/25 -> RoadLinesPolynoms[100000]/roadLinesPolynomsArray[3]/lineId/1
  Demux/24 -> RoadLinesPolynoms[100000]/roadLinesPolynomsArray[2]/estimatedCurvatureRadius/1
  Demux/23 -> RoadLinesPolynoms[100000]/roadLinesPolynomsArray[2]/curvatureRadius/1
  Demux/22 -> RoadLinesPolynoms[100000]/roadLinesPolynomsArray[2]/c3/1
  Demux/21 -> RoadLinesPolynoms[100000]/roadLinesPolynomsArray[2]/c2/1
  Demux/20 -> RoadLinesPolynoms[100000]/roadLinesPolynomsArray[2]/c1/1
  Demux/19 -> RoadLinesPolynoms[100000]/roadLinesPolynomsArray[2]/c0/1
  Demux/18 -> RoadLinesPolynoms[100000]/roadLinesPolynomsArray[2]/lineId/1
  Demux/17 -> RoadLinesPolynoms[100000]/roadLinesPolynomsArray[1]/estimatedCurvatureRadius/1
  Demux/16 -> RoadLinesPolynoms[100000]/roadLinesPolynomsArray[1]/curvatureRadius/1
  Demux/15 -> RoadLinesPolynoms[100000]/roadLinesPolynomsArray[1]/c3/1
  Demux/14 -> RoadLinesPolynoms[100000]/roadLinesPolynomsArray[1]/c2/1
  Demux/13 -> RoadLinesPolynoms[100000]/roadLinesPolynomsArray[1]/c1/1
  Demux/12 -> RoadLinesPolynoms[100000]/roadLinesPolynomsArray[1]/c0/1
  Demux/11 -> RoadLinesPolynoms[100000]/roadLinesPolynomsArray[1]/lineId/1
  Demux/10 -> RoadLinesPolynoms[100000]/roadLinesPolynomsArray[0]/estimatedCurvatureRadius/1
  Demux/9 -> RoadLinesPolynoms[100000]/roadLinesPolynomsArray[0]/curvatureRadius/1
  Demux/8 -> RoadLinesPolynoms[100000]/roadLinesPolynomsArray[0]/c3/1
  Demux/7 -> RoadLinesPolynoms[100000]/roadLinesPolynomsArray[0]/c2/1
  Demux/6 -> RoadLinesPolynoms[100000]/roadLinesPolynomsArray[0]/c1/1
  Demux/5 -> RoadLinesPolynoms[100000]/roadLinesPolynomsArray[0]/c0/1
  Demux/4 -> RoadLinesPolynoms[100000]/roadLinesPolynomsArray[0]/lineId/1
  Demux/3 -> VehicleUpdate[0]/roadInfo[0]/laneGap/1
  Demux/2 -> VehicleUpdate[0]/roadInfo[0]/roadAngle/1
  Demux/1 -> VehicleUpdate[0]/roadInfo[0]/roadAbscissa/1
  UDP Receive/1 -> Switch/1

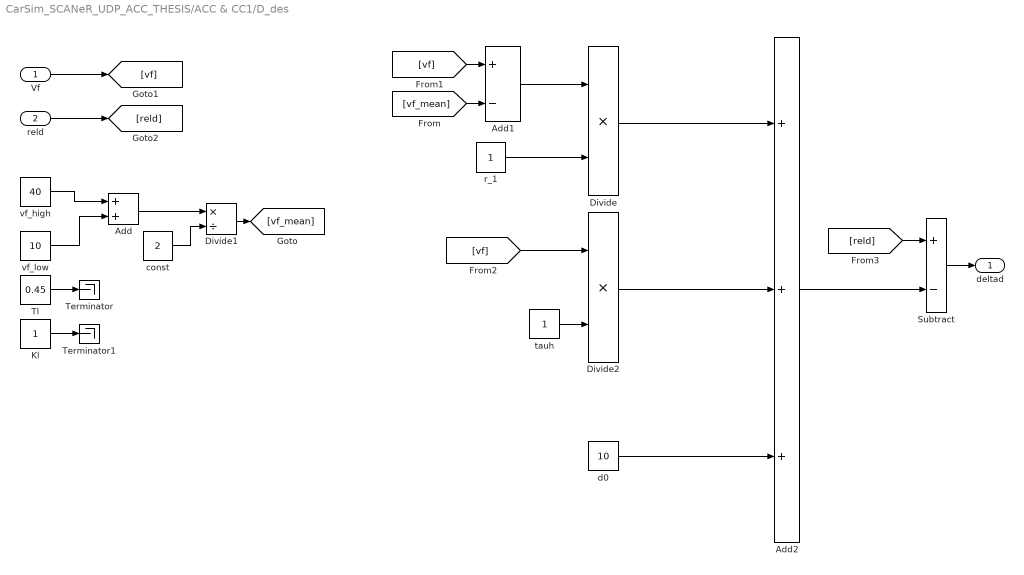
== system CarSim_SCANeR_UDP_ACC_THESIS/ACC & CC1/D_des ==
  "Vf " : Inport
  reld : Inport  Port=2
  Add : Sum
  Add1 : Sum  Inputs=+-
  Add2 : Sum  Inputs=+++
  Divide : Product  Inputs=**
  Divide1 : Product  Inputs=*/
  Divide2 : Product  Inputs=**
  Kl : Constant
  Subtract : Sum  Inputs=+-
  Terminator : Terminator
  Terminator1 : Terminator
  Tl : Constant  Value=0.45
  const : Constant  Value=2
  d0 : Constant  Value=10
  "r_1 " : Constant
  "tauh " : Constant
  vf_high : Constant  Value=40
  vf_low : Constant  Value=10
  deltad : Outport
  wires:
  Subtract/1 -> deltad/1
  [reld] -> Subtract/1
  Add2/1 -> Subtract/2
  reld/1 -> [reld]
  Kl/1 -> Terminator1/1
  Tl/1 -> Terminator/1
  d0/1 -> Add2/3
  Divide2/1 -> Add2/2
  Divide/1 -> Add2/1
  "tauh "/1 -> Divide2/2
  [vf] -> Divide2/1
  [vf] -> Add1/1
  "Vf "/1 -> [vf]
  "r_1 "/1 -> Divide/2
  Add1/1 -> Divide/1
  [vf_mean] -> Add1/2
  Divide1/1 -> [vf_mean]
  const/1 -> Divide1/2
  Add/1 -> Divide1/1
  vf_low/1 -> Add/2
  vf_high/1 -> Add/1

== system CarSim_SCANeR_UDP_ACC_THESIS/ACC & CC1/D_des1 ==
  "Vf " : Inport
  reld : Inport  Port=2
  D_des_sfcn : S-Function  FunctionName=D_des_sf  SFunctionModules=""  SFunctionDeploymentMode=off  EnableBusSupport=off  mask{rtw_sf_name=D_des_sf, showVar=off}
      mask prompts: rtw_sf_name "Simulink:masks:GenSFuncName_MP"; showVar "Simulink:masks:GenSFuncShowModuleList_MP"
      mask help: Simulink:masks:GenSFuncDesc_MD
      mask init:
      | displist = '';
      | if ~strcmp(get_param(gcb, 'FunctionName'), rtw_sf_name);
      |   set_param(gcb, 'FunctionName', rtw_sf_name);
      | end
      | % Check if we are generating code
      | rtw_mode = false;
      | if strcmpi(get_param(bdroot(gcb),'SimulationStatus'),'Initializing')
      | 	rtw_mode = strcmpi(get_param(bdroot(gcb),'BuildingRTWCode'),'on') && ...
      | 		~strcmpi(get_param(bdroot(gcb),'TargetStyle'),'SimulationTarget');
      | end
      | if showVar || rtw_mode
      | 	if exist('rtwsfunc') == 2 | exist('rtwsfunc') == 6
      | 		tmplist = rtwsfunc(rtw_sf_name,gcb);
      | 		tmplist = DAStudio.message('Simulink:masks:GenSFuncListOfModules_IC', tmplist);
      | 	elseif showVar
      | 		tmplist1 = DAStudio.message('Simulink:masks:GenSFuncListOfModules_IC', '');
      |         tmplist2 = DAStudio.message('Simulink:masks:GenSFuncNotLicensed_IC');
      |         tmplist = [tmplist1 tmplist2];
      |  	end
      | end
      | if showVar
      |   displist = tmplist;
      | end
      settings: CopyFcn=|
      | if ~strcmp(get_param(gcb,'Linkstatus'),'none') && ...
      | ~strcmp(get_param(gcb,'Linkstatus'),'implicit')
      |   set_param(gcb,'LinkStatus','none');
      | end
      mask Help: eval('feval(''rtwprivate'',''rtwhelpview'',''rtw_sfcn_block'')');
      mask Display:
      | port_label('input',1,'Vf ');
      | port_label('input',2,'reld');
      | port_label('output',1,'deltad');
  __InputSSForSFun__ : Subsystem
  __OutputSSForSFun__ : Subsystem
  deltad : Outport
  wires:
  __OutputSSForSFun__/1(deltad) -> deltad/1
  D_des_sfcn/1 -> __OutputSSForSFun__/1(__UniqueInportName__1__)
  __InputSSForSFun__/2(__UniqueOutportName__2__) -> D_des_sfcn/2
  __InputSSForSFun__/1(__UniqueOutportName__1__) -> D_des_sfcn/1
  reld/1 -> __InputSSForSFun__/2(reld)
  "Vf "/1 -> __InputSSForSFun__/1("Vf ")

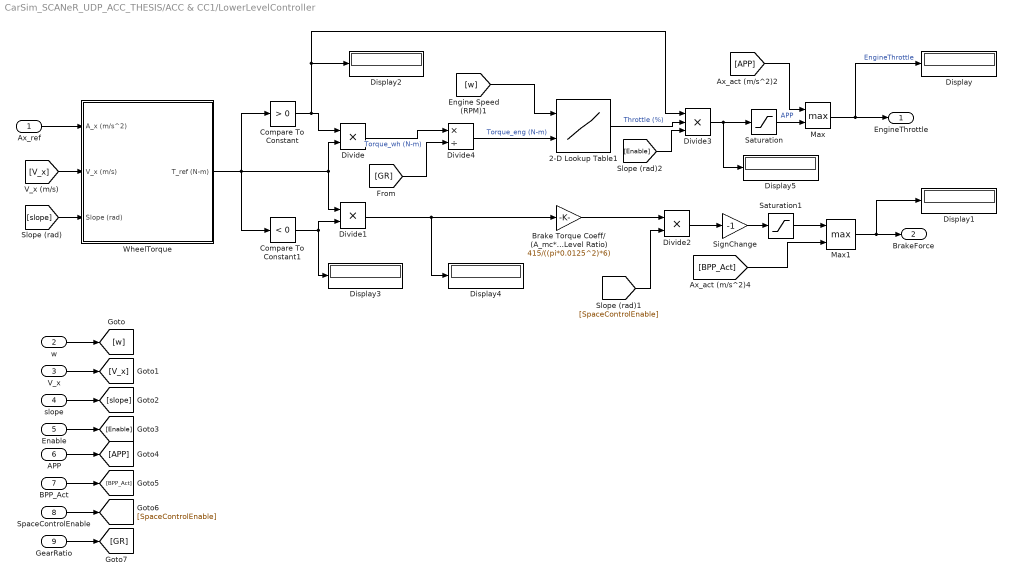
== system CarSim_SCANeR_UDP_ACC_THESIS/ACC & CC1/LowerLevelController ==
  Ax_ref : Inport
  w : Inport  Port=2
  V_x : Inport  Port=3
  slope : Inport  Port=4
  Enable : Inport  Port=5
  APP : Inport  Port=6
  BPP_Act : Inport  Port=7
  SpaceControlEnable : Inport  Port=8
  GearRatio : Inport  Port=9
  2-D Lookup Table1 : Lookup_n-D  BreakpointsForDimension1=[0,750,1000,1500,2000,3000,4000,5000,6000,6500,7000,7500,7550,7600,7700,7900,8500]  BreakpointsForDimension2=[-93,-46.5,0,46.5,93,139.5,186,232.5,279,325.5,372,418.5]  Table=reshape([0,0,0,0,0,0,0,0,0,0,0,0,0,0,0,0,0,0,0,0,0,0,0,0,0.0099,0.0185,0.0185,0.026,0.0315,0,0,0,0,0,0,0,0,0.0067,0.0192,0.0288,0.0357,0.0428,0.0494,0.0494,0.0549,0.0664,0,0,0,0,0,0,0.1281,0.1194,0.0733,0.0673,0.0699,0.0714,0.0757,0.0802,0.0802,0.0838,0.1017,0,0,0,0,0,0,0.4500,0.3444,0.1214,0.1095,0.1077,0.1056,0.1075,0.1110,0.1110,0.1141,0.1448,0,0,0,0,0,0,0.9375,0.8333,0.1857,0.1393,0.1366,0.1333,0.1362,0.1415,0.1415,0.1462,0.3397,0,0,0,0,0,0,1,1,0.3643,0.2452,0.2274,0.2056,0.2247,0.2598,0.2598,0.3397,0.6483,0,0,0,0,0,0,1,1,0.6286,0.3940,0.3717,0.3444,0.3684,0.4195,0.4195,0.5846,0.9167,0,0,0,0,0,0,1,1,0.8571,0.6286,.5857,0.5333,0.5793,0.6634,0.6634,0.8172,1,0,0,0,0,0,0,1,1,1,0.8333,.8083,0.7556,0.8046,0.8537,0.8537,0.9247,1,0,0,0,0,0,0,1,1,1,0.9524,0.9238,0.8898,0.9195,.9756,0.9756,1,1,0,0,0,0,0,0,1,1,1,1,1,1,1,1,1,1,1,0,0,0,0,0],17,12)  InternalRulePriority=Speed  RndMeth=Simplest  InputSameDT=on
  Brake Torque Coeff/ (A_mc*Pedal Level Ratio) : Gain  Gain=415/((pi*0.0125^2)*6)
  Compare To Constant : simulink/Logic and Bit Operations/Compare To Constant  relop=>  const=0  OutDataTypeStr=boolean
  Compare To Constant1 : simulink/Logic and Bit Operations/Compare To Constant  relop=<  const=0  OutDataTypeStr=boolean
  Display{,1..5} (6 alike) : Display
  Divide : Product  Inputs=**
  Divide1 : Product  Inputs=**
  Divide2 : Product  Inputs=**
  Divide3 : Product  Inputs=***
  Divide4 : Product  Inputs=*/
  Max : MinMax  Function=max  Inputs=2
  Max1 : MinMax  Function=max  Inputs=2
  Saturation : Saturate  UpperLimit=1  LowerLimit=0
  Saturation1 : Saturate  UpperLimit=200  LowerLimit=0
  SignChange : Gain  Gain=-1
  WheelTorque : Subsystem
      settings: AttributesFormatString=Name='abc'
  EngineThrottle : Outport
  BrakeForce : Outport  Port=2
  wires:
  Divide/1 -> Divide4/1  "Torque_wh (N-m)"
  [GR] -> Divide4/2
  GearRatio/1 -> [GR]
  SpaceControlEnable/1 -> [SpaceControlEnable]
  BPP_Act/1 -> [BPP_Act]
  APP/1 -> [APP]
  Enable/1 -> [Enable]
  slope/1 -> [slope]
  V_x/1 -> [V_x]
  w/1 -> [w]
  Max1/1 -> Display1/1, BrakeForce/1
  Saturation/1 -> Max/2  "APP"
  Compare To Constant1/1 -> Display3/1, Divide1/2
  [w] -> 2-D Lookup Table1/1
  Saturation1/1 -> Max1/1
  [BPP_Act] -> Max1/2
  Divide2/1 -> SignChange/1
  Divide3/1 -> Display5/1, Saturation/1
  Compare To Constant/1 -> Divide3/1, Display2/1, Divide/1
  Max/1 -> Display/1, EngineThrottle/1  "EngineThrottle"
  [SpaceControlEnable] -> Divide2/2
  SignChange/1 -> Saturation1/1
  [slope] -> WheelTorque/3(Slope (rad))
  [V_x] -> WheelTorque/2(V_x (m/s))
  WheelTorque/1(T_ref (N-m)) -> Divide1/1, Divide/2, Compare To Constant/1, Compare To Constant1/1
  Divide1/1 -> Display4/1, Brake Torque Coeff/ (A_mc*Pedal Level Ratio)/1
  Ax_ref/1 -> WheelTorque/1(A_x (m/s^2))
  Divide4/1 -> 2-D Lookup Table1/2  "Torque_eng (N-m)"
  Brake Torque Coeff/ (A_mc*Pedal Level Ratio)/1 -> Divide2/1
  2-D Lookup Table1/1 -> Divide3/2  "Throttle (%)"
  [APP] -> Max/1
  [Enable] -> Divide3/3
